simulink model "Day1_model2"  (R2022b)
settings: Solver=ode4  StartTime=0.0  StopTime=10.0  FixedStep=0.001  RelTol=1e-3
values from neighbouring files (symbols this model uses):
  C = 0.1    [Day1_2.m]
  freq = 1    [Day1_2.m]
  L = 2    [Day1_2.m]
  R = 30    [Day1_2.m]
settings Model: Creator=user  LastModifiedBy=user

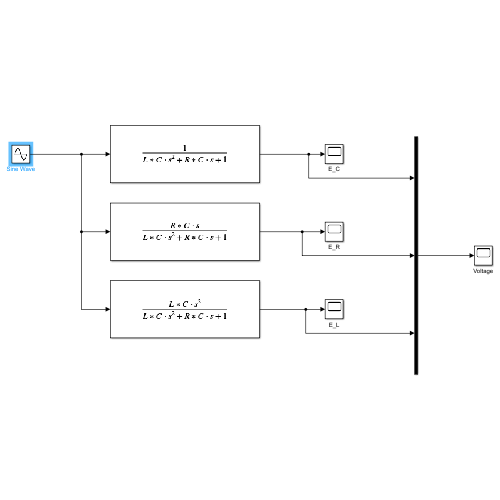
[thumbnail: Simulink's stored preview of the top-level diagram]
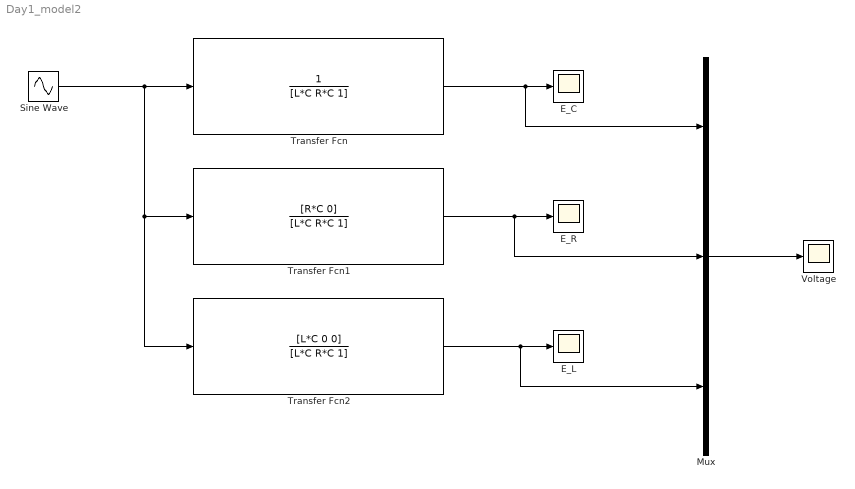
== system Day1_model2 ==
  E_C : Scope
  E_L : Scope
  E_R : Scope
  Mux : Mux  Inputs=3
  Sine Wave : Sin  Frequency=freq*2*pi  SampleTime=0
  Transfer Fcn : TransferFcn  Denominator=[L*C R*C 1]
  Transfer Fcn1 : TransferFcn  Numerator=[R*C 0]  Denominator=[L*C R*C 1]
  Transfer Fcn2 : TransferFcn  Numerator=[L*C 0 0]  Denominator=[L*C R*C 1]
  Voltage : Scope
  wires:
  Transfer Fcn/1 -> Mux/1, E_C/1
  Transfer Fcn1/1 -> Mux/2, E_R/1
  Transfer Fcn2/1 -> Mux/3, E_L/1
  Mux/1 -> Voltage/1
  Sine Wave/1 -> Transfer Fcn2/1, Transfer Fcn1/1, Transfer Fcn/1
